simulink model "mower_model"  (R2018b)
settings: Solver=VariableStepAuto  StartTime=0.0  StopTime=10.0  RelTol=1e-3
settings Model: Creator=filipkronstrom  LastModifiedBy=filipkronstrom

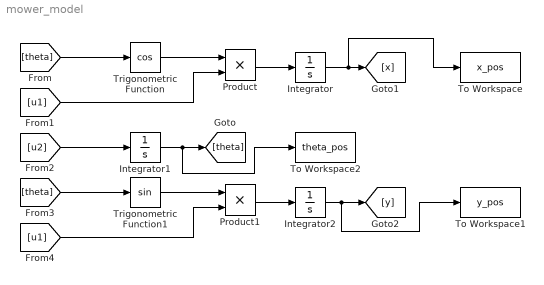
== system mower_model ==
  Integrator : Integrator
  Integrator1 : Integrator
  Integrator2 : Integrator
  Product : Product
  Product1 : Product
  To Workspace : ToWorkspace  VariableName=x_pos  SaveFormat=Timeseries  SampleTime=-1
  To Workspace1 : ToWorkspace  VariableName=y_pos  SaveFormat=Timeseries  SampleTime=-1
  To Workspace2 : ToWorkspace  VariableName=theta_pos  SaveFormat=Timeseries  SampleTime=-1
  Trigonometric Function : Trigonometry  Operator=cos
  Trigonometric Function1 : Trigonometry
  wires:
  Trigonometric Function/1 -> Product/1
  Product/1 -> Integrator/1
  Integrator1/1 -> To Workspace2/1, [theta]
  [theta] -> Trigonometric Function/1
  [u1] -> Product/2
  [u2] -> Integrator1/1
  [theta] -> Trigonometric Function1/1
  Trigonometric Function1/1 -> Product1/1
  [u1] -> Product1/2
  Product1/1 -> Integrator2/1
  Integrator/1 -> To Workspace/1, [x]
  Integrator2/1 -> To Workspace1/1, [y]
